simulink model "assignment_3_simulink"  (R2024a)
settings: Solver=ode23t  StartTime=0.0  StopTime=200  MaxStep=1e-4  RelTol=1e-3
values from neighbouring files (symbols this model uses):
  A = [a_11 a_12 a_13 a_14 ... (first row only)    [assignment_3.m]
  B_1 = [b1_1; b1_2; b1_3; b1_4]    [assignment_3.m]
  B_2 = [b2_1; b2_2; b2_3; b2_4]    [assignment_3.m]
  C = eye(4)    [assignment_3.m]
  delta_constraint = deg2rad(25)    [assignment_3.m]
  K_ff = (m_v*V_x^2/l)*(l_r/C_f-l_f/C_r+(l_f/C_r)*K(3))+l-l_r*K(3)    [assignment_3.m]
  V_x = 22.2    [assignment_3.m]
undefined symbols (not defined in the file or in its folder): K
settings Model: Creator=erlendskinnemoen  LastModifiedBy=fjmo

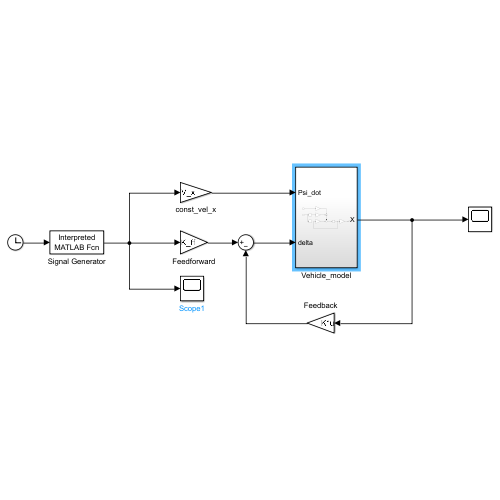
[thumbnail: Simulink's stored preview of the top-level diagram]
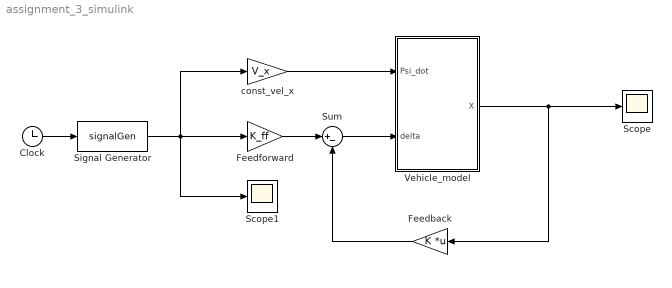
== system assignment_3_simulink ==
  Clock : Clock
  Feedback : Gain  Gain=K  Multiplication=Matrix(K*u)
  Feedforward : Gain  Gain=K_ff
  Scope : Scope
  Scope1 : Scope
  Signal Generator : MATLABFcn  MATLABFcn=signalGen
  Sum : Sum  Inputs=|+-
  Vehicle_model : Subsystem
  const_vel_x : Gain  Gain=V_x
  wires:
  Feedback/1 -> Sum/2
  Sum/1 -> Vehicle_model/2(delta)
  Feedforward/1 -> Sum/1
  Vehicle_model/1(X) -> Feedback/1, Scope/1
  Clock/1 -> Signal Generator/1
  Signal Generator/1 -> Scope1/1, const_vel_x/1, Feedforward/1
  const_vel_x/1 -> Vehicle_model/1(Psi_dot)

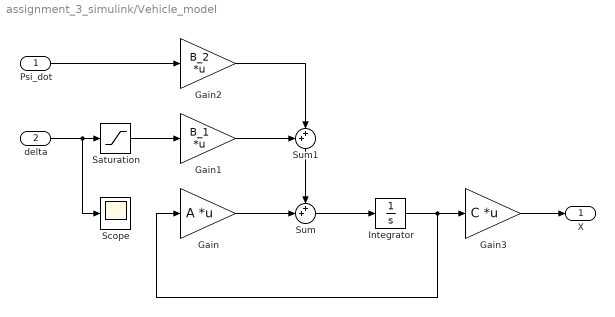
== system assignment_3_simulink/Vehicle_model ==
  Psi_dot : Inport
  delta : Inport  Port=2
  Gain : Gain  Gain=A  Multiplication=Matrix(K*u)
  Gain1 : Gain  Gain=B_1  Multiplication=Matrix(K*u)
  Gain2 : Gain  Gain=B_2  Multiplication=Matrix(K*u)
  Gain3 : Gain  Gain=C  Multiplication=Matrix(K*u)
  Integrator : Integrator
  Saturation : Saturate  UpperLimit=delta_constraint  LowerLimit=-delta_constraint
  Scope : Scope
  Sum : Sum  Inputs=++|
  Sum1 : Sum  Inputs=++|
  X : Outport
  wires:
  Integrator/1 -> Gain3/1, Gain/1
  Psi_dot/1 -> Gain2/1
  delta/1 -> Scope/1, Saturation/1
  Saturation/1 -> Gain1/1
  Gain2/1 -> Sum1/2
  Gain1/1 -> Sum1/1
  Sum1/1 -> Sum/1
  Gain/1 -> Sum/2
  Sum/1 -> Integrator/1
  Gain3/1 -> X/1
